simulink subsystem "data_logging_for_lead_veh_subsystem"  (R2025a)
settings: Solver=VariableStepAuto  StartTime=0.0  StopTime=10.0  RelTol=1e-3
settings Model: Creator=admin  LastModifiedBy=admin

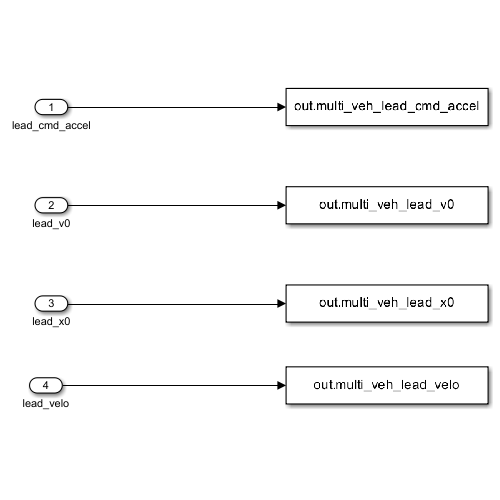
[thumbnail: Simulink's stored preview of the top-level diagram]
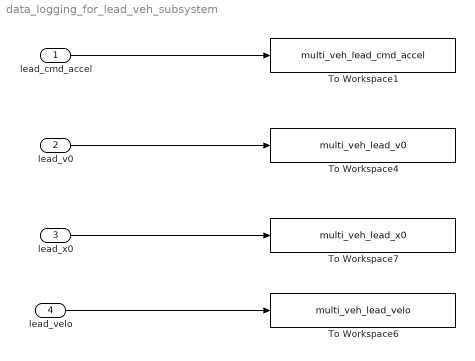
== system data_logging_for_lead_veh_subsystem ==
  lead_cmd_accel : Inport
  lead_v0 : Inport  Port=2
  lead_x0 : Inport  Port=3
  lead_velo : Inport  Port=4
  To Workspace1 : ToWorkspace  VariableName=multi_veh_lead_cmd_accel  SaveFormat=Structure With Time  SampleTime=-1
  To Workspace4 : ToWorkspace  VariableName=multi_veh_lead_v0  SaveFormat=Structure With Time  SampleTime=-1
  To Workspace6 : ToWorkspace  VariableName=multi_veh_lead_velo  SaveFormat=Structure With Time  SampleTime=-1
  To Workspace7 : ToWorkspace  VariableName=multi_veh_lead_x0  SaveFormat=Structure With Time  SampleTime=-1
  wires:
  lead_velo/1 -> To Workspace6/1
  lead_v0/1 -> To Workspace4/1
  lead_cmd_accel/1 -> To Workspace1/1
  lead_x0/1 -> To Workspace7/1
